simulink model "VOO"  (R2022b)
settings: Solver=FixedStepAuto  StartTime=0.0  StopTime=10.0  FixedStep=1e-3  RelTol=1e-3  EnableMultiTasking=on
undefined symbols (not defined in the file): D10, D11, D12, D2, D4, D5, D7, D8, D9, PTA0, PTA2, PTB23, PTB9, PTC3, PTC4, PTD0, PTD2, PTD3
libraries: frdmk64flib x9
settings Model: ExtModeTrigDuration=5  Creator=16475  LastModifiedBy=16475
settings OptimizationCC: EnhancedBackFolding=on  PassReuseOutputArgsAs=Individual arguments  ZeroExternalMemoryAtStartup=off  ZeroInternalMemoryAtStartup=off  MaxStackSize=64  OptimizeBlockOrder=speed  DifferentSizesBufferReuse=on  OptimizationCustomize=off  EfficientTunableParamExpr=on
settings DebuggingCC: ParameterTunabilityLossMsg=error
settings HardwareCC: ProdBitPerPointer=32  ProdBitPerSizeT=32  ProdBitPerPtrDiffT=32  ProdLargestAtomicInteger=Long  ProdLargestAtomicFloat=Double  ProdWordSize=32  ProdHWDeviceType=ARM Compatible->ARM Cortex
settings SFSimCC: MATLABDynamicMemAlloc=off
settings RTWCC: Description=Embedded Coder  SystemTargetFile=ert.tlc  HardwareBoard=NXP FRDM-K64F  TLCOptions="-aInlineSetEventsForThisBaseRateFcn=TLC_FALSE -aSuppressMultiTaskScheduler=TLC_FALSE  -aRateBasedStepFcn=0"  TemplateMakefile=ert_default_tmf  Toolchain=GNU Tools for ARM Embedded Processors
settings CodeAppCC: ForceParamTrailComments=on  IgnoreCustomStorageClasses=off  OperatorAnnotations=on  SimulinkDataObjDesc=on  SFDataObjDesc=on  InsertBlockDesc=on
settings ERTTargetCC: ExtModeTransport=4  ExtModeMexFile=sendToCommService

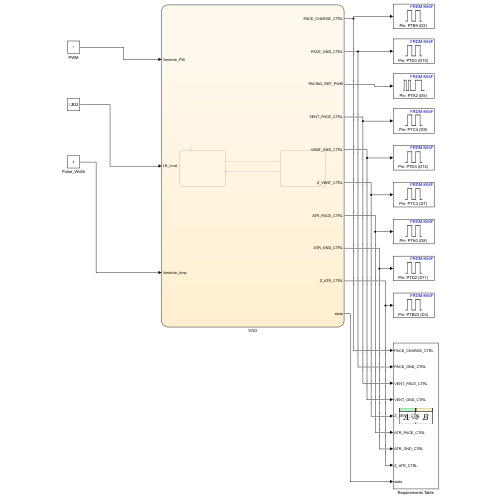
[thumbnail: Simulink's stored preview of the top-level diagram]
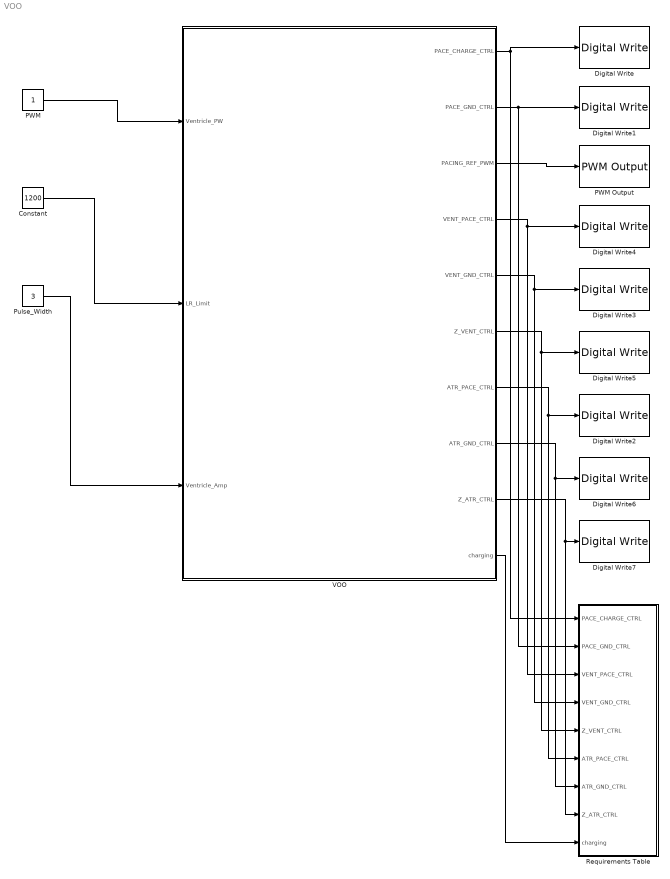
== system VOO ==
  Constant : Constant  Value=1200
  Digital Write : frdmk64flib/Digital Write  Whichpin=PTB9 (D2)
  Digital Write1 : frdmk64flib/Digital Write  Whichpin=PTD0 (D10)
  Digital Write2 : frdmk64flib/Digital Write  Whichpin=PTA0 (D8)
  Digital Write3 : frdmk64flib/Digital Write  Whichpin=PTD3 (D12)
  Digital Write4 : frdmk64flib/Digital Write  Whichpin=PTC4 (D9)
  Digital Write5 : frdmk64flib/Digital Write  Whichpin=PTC3 (D7)
  Digital Write6 : frdmk64flib/Digital Write  Whichpin=PTD2 (D11)
  Digital Write7 : frdmk64flib/Digital Write  Whichpin=PTB23 (D4)
  PWM : Constant
  PWM Output : frdmk64flib/PWM Output  Whichpin=PTA2 (D5)  InitialFrequency=2000  InitialDutyCycle=0
  Pulse_Width : Constant  Value=3
  Requirements Table : Requirements Table  TreatAsAtomicUnit=on
  VOO : Stateflow chart  TreatAsAtomicUnit=on
      settings: PortSchema="{\"entries\":[{\"content\":{\"sides\":[{\"content\":{\"connectorIds\":[\"In1\",\"In2\",\"In3\"]},\"type\":\"ConnectorPlacement.EquallySpacedRectSide\",\"uuid\":\"a3e94f58-3093-42a5-91db-f56c9d127bee\"},{\"content\":{\"connectorIds\":[\"Out1\",\"Out2\",\"Out3\",\"Out5\",\"Out4\",\"Out7\",\"Out6\",\"Out8\",\"Out9\",\"Out10\"],\"side\":\"RIGHT\"},\"type\":\"ConnectorPlacement.EquallySpacedRectSide\",\"uuid\":\"289ad049-9840-4721-af22-1385d5696f7c\"},{\"content\":{\"connectorIds\":[],\"side\":\"TOP\"},\"type\":\"ConnectorPlacement.EquallySpacedRectSide\",\"uuid\":\"4602f2ad-cb91-4c7a-9db6-6571445db01f\"}]},\"type\":\"ConnectorPlacement.EquallySpacedConnector\",\"uuid\":\"bfd50937-4990-4c1b-ba87-ff4dc7d3240f\"}],\"packageUris\":[\"http://schema.mathworks.com/mf0/Connector/R2020b\"],\"version\":\"1.0\"}"
  wires:
  VOO/3(PACING_REF_PWM) -> PWM Output/1
  Pulse_Width/1 -> VOO/3(Ventricle_Amp)
  PWM/1 -> VOO/1(Ventricle_PW)
  Constant/1 -> VOO/2(LR_Limit)
  VOO/8(ATR_GND_CTRL) -> Requirements Table/7(ATR_GND_CTRL), Digital Write6/1
  VOO/6(ATR_PACE_CTRL) -> Requirements Table/6(ATR_PACE_CTRL), Digital Write2/1
  VOO/1(PACE_CHARGE_CTRL) -> Requirements Table/1(PACE_CHARGE_CTRL), Digital Write/1
  VOO/4(VENT_GND_CTRL) -> Requirements Table/4(VENT_GND_CTRL), Digital Write3/1
  VOO/7(Z_VENT_CTRL) -> Requirements Table/5(Z_VENT_CTRL), Digital Write5/1
  VOO/9(Z_ATR_CTRL) -> Requirements Table/8(Z_ATR_CTRL), Digital Write7/1
  VOO/5(VENT_PACE_CTRL) -> Requirements Table/3(VENT_PACE_CTRL), Digital Write4/1
  VOO/2(PACE_GND_CTRL) -> Requirements Table/2(PACE_GND_CTRL), Digital Write1/1
  VOO/10(charging) -> Requirements Table/9(charging)

== stateflow chart VOO/VOO ==
  state Charging_C22
    entry:
    ATR_PACE_CTRL = false;
    VENT_PACE_CTRL = false;
    PACING_REF_PWM = ((Ventricle_Amp/5)*100);
    PACE_CHARGE_CTRL = true;
    PACE_GND_CTRL = true;
    Z_ATR_CTRL = false;
    Z_VENT_CTRL = false;
    ATR_GND_CTRL = false;
    VENT_GND_CTRL = true;
    charging = true;
  state Discharging_C22
    entry:
    PACE_CHARGE_CTRL = false;
    PACE_GND_CTRL = true;
    ATR_PACE_CTRL = false;
    VENT_PACE_CTRL = true;
    Z_ATR_CTRL = false;
    Z_VENT_CTRL = false;
    ATR_GND_CTRL = false;
    VENT_GND_CTRL = false;
    charging = false;
  (default) -> Charging_C22
  Charging_C22 -> Discharging_C22 : [after(LR_Limit - Ventricle_PW,msec)]
  Discharging_C22 -> Charging_C22 : [after(Ventricle_PW,msec)]
  data: Ventricle_PW input double; LR_Limit input double; PACE_CHARGE_CTRL output boolean; PACE_GND_CTRL output boolean; PACING_REF_PWM output double; VENT_GND_CTRL output boolean; VENT_PACE_CTRL output boolean; ATR_PACE_CTRL output boolean; Z_VENT_CTRL output boolean; Ventricle_Amp input double; ATR_GND_CTRL output boolean; Z_ATR_CTRL output boolean; charging output

== stateflow chart VOO/Requirements Table ==
  (default) -> (junction 1073742576)
  (junction 1073742576) -> (junction 1073742577) : {
      | % SF_REQ_REV_07
      | }
  (junction 1073742577) -> (junction 1073742579) : {
      | % HEADER_ASSIGNMENTS
      |
      | }
  (junction 1073742579) -> (junction 1073742581) : {
      | % START_A_4
      | }
  (junction 1073742581) -> (junction 1073742583) : {
      | }
  (junction 1073742583) -> (junction 1073742585)
  (junction 1073742585) -> (junction 1073742587) : {
      | }
  (junction 1073742587) -> (junction 1073742589) : {
      | % END_A_4
      | }
  (junction 1073742589) -> (junction 1073742591) : {
      | % START_R_1
      | }
  (junction 1073742591) -> (junction 1073742593) : {
      | }
  (junction 1073742593) -> (junction 1073742595)
  (junction 1073742595) -> (junction 1073742597) [order 1] : [(((prev(charging)) == (prev(charging) == false)))]
  (junction 1073742595) -> (junction 1073742603) [order 2]
  (junction 1073742597) -> (junction 1073742599) : {
      | reqtable_postcondition((((PACE_CHARGE_CTRL) == (true))) && (((PACE_GND_CTRL) == (true))) && (((VENT_PACE_CTRL) == (false))) && (((VENT_GND_CTRL) == (true))) && (((Z_VENT_CTRL) == (false))) && (((ATR_PACE_CTRL) == (false))) && (((ATR_GND_CTRL) == (false))) && (((Z_ATR_CTRL) == (false))) && (((charging) == (true))), 'R:1');
      |
      |
      | }
  (junction 1073742599) -> (junction 1073742601) : {
      | }
  (junction 1073742601) -> (junction 1073742603)
  (junction 1073742603) -> (junction 1073742605)
  (junction 1073742605) -> (junction 1073742607) : {
      | % END_R_1
      | }
  (junction 1073742607) -> (junction 1073742609) : {
      | % START_R_7
      | }
  (junction 1073742609) -> (junction 1073742611) : {
      | }
  (junction 1073742611) -> (junction 1073742613)
  (junction 1073742613) -> (junction 1073742615) [order 1] : [(((prev(charging)) == (prev(charging) == true)))]
  (junction 1073742613) -> (junction 1073742621) [order 2]
  (junction 1073742615) -> (junction 1073742617) : {
      | reqtable_postcondition((((PACE_CHARGE_CTRL) == (false))) && (((PACE_GND_CTRL) == (true))) && (((VENT_PACE_CTRL) == (true))) && (((VENT_GND_CTRL) == (false))) && (((Z_VENT_CTRL) == (false))) && (((ATR_PACE_CTRL) == (false))) && (((ATR_GND_CTRL) == (false))) && (((Z_ATR_CTRL) == (false))) && (((charging) == (false))), 'R:2');
      |
      |
      | }
  (junction 1073742617) -> (junction 1073742619) : {
      | }
  (junction 1073742619) -> (junction 1073742621)
  (junction 1073742621) -> (junction 1073742623)
  (junction 1073742623) -> (junction 1073742625) : {
      | % END_R_7
      | }
  data: PACE_CHARGE_CTRL input boolean; PACE_GND_CTRL input boolean; VENT_PACE_CTRL input boolean; VENT_GND_CTRL input boolean; Z_VENT_CTRL input boolean; ATR_PACE_CTRL input boolean; ATR_GND_CTRL input boolean; Z_ATR_CTRL input boolean; charging input boolean
